simulink model "CM020A_Bmw5441McuCfg"  (R2013b)
settings: Solver=FixedStepDiscrete  SolverMode=SingleTasking  StartTime=0.0  StopTime=1  FixedStep=0.0005  RelTol=1e-3
PreLoadFcn:
  | CM020A_Bmw5441McuCfg_DataDict
values from neighbouring files (symbols this model uses):
  ADC0CFGANDUSE_ADCD0SGVCEP2_CNT_U08 = DataDict.Constant    [CM020A_Bmw5441McuCfg_DataDict.m]
  ADC0CFGANDUSE_ADCD0SGVCEP3_CNT_U08 = DataDict.Constant    [CM020A_Bmw5441McuCfg_DataDict.m]
  ADC0CFGANDUSE_ADCD0SGVCSP2_CNT_U08 = DataDict.Constant    [CM020A_Bmw5441McuCfg_DataDict.m]
  ADC0CFGANDUSE_ADCD0SGVCSP3_CNT_U08 = DataDict.Constant    [CM020A_Bmw5441McuCfg_DataDict.m]
  ADC0CFGANDUSE_ADCD0VCR00_CNT_U32 = DataDict.Constant    [CM020A_Bmw5441McuCfg_DataDict.m]
  ADC0CFGANDUSE_ADCD0VCR01_CNT_U32 = DataDict.Constant    [CM020A_Bmw5441McuCfg_DataDict.m]
  ADC0CFGANDUSE_ADCD0VCR02_CNT_U32 = DataDict.Constant    [CM020A_Bmw5441McuCfg_DataDict.m]
  ADC0CFGANDUSE_ADCD0VCR03_CNT_U32 = DataDict.Constant    [CM020A_Bmw5441McuCfg_DataDict.m]
  ADC0CFGANDUSE_ADCD0VCR04_CNT_U32 = DataDict.Constant    [CM020A_Bmw5441McuCfg_DataDict.m]
  ADC0CFGANDUSE_ADCD0VCR05_CNT_U32 = DataDict.Constant    [CM020A_Bmw5441McuCfg_DataDict.m]
  ADC0CFGANDUSE_ADCD0VCR06_CNT_U32 = DataDict.Constant    [CM020A_Bmw5441McuCfg_DataDict.m]
  ADC0CFGANDUSE_ADCD0VCR07_CNT_U32 = DataDict.Constant    [CM020A_Bmw5441McuCfg_DataDict.m]
  ADC0CFGANDUSE_ADCD0VCR08_CNT_U32 = DataDict.Constant    [CM020A_Bmw5441McuCfg_DataDict.m]
  ADC0CFGANDUSE_ADCD0VCR09_CNT_U32 = DataDict.Constant    [CM020A_Bmw5441McuCfg_DataDict.m]
  ADC0CFGANDUSE_ADCD0VCR10_CNT_U32 = DataDict.Constant    [CM020A_Bmw5441McuCfg_DataDict.m]
  ADC0CFGANDUSE_ADCD0VCR11_CNT_U32 = DataDict.Constant    [CM020A_Bmw5441McuCfg_DataDict.m]
  ADC0CFGANDUSE_ADCD0VCR12_CNT_U32 = DataDict.Constant    [CM020A_Bmw5441McuCfg_DataDict.m]
  ADC0CFGANDUSE_ADCD0VCR13_CNT_U32 = DataDict.Constant    [CM020A_Bmw5441McuCfg_DataDict.m]
  ADC0CFGANDUSE_ADCD0VCR14_CNT_U32 = DataDict.Constant    [CM020A_Bmw5441McuCfg_DataDict.m]
  ADC0CFGANDUSE_ADCD0VCR15_CNT_U32 = DataDict.Constant    [CM020A_Bmw5441McuCfg_DataDict.m]
  ADC0CFGANDUSE_ADCD0VCR16_CNT_U32 = DataDict.Constant    [CM020A_Bmw5441McuCfg_DataDict.m]
  ADC0CFGANDUSE_ADCD0VCR17_CNT_U32 = DataDict.Constant    [CM020A_Bmw5441McuCfg_DataDict.m]
  ADC0CFGANDUSE_ADCD0VCR18_CNT_U32 = DataDict.Constant    [CM020A_Bmw5441McuCfg_DataDict.m]
  ADC0CFGANDUSE_ADCD0VCR19_CNT_U32 = DataDict.Constant    [CM020A_Bmw5441McuCfg_DataDict.m]
  ADC0CFGANDUSE_ADCD0VCR20_CNT_U32 = DataDict.Constant    [CM020A_Bmw5441McuCfg_DataDict.m]
  ADC0CFGANDUSE_ADCSCAGFAC_VOLTPERCNT_F32 = DataDict.Constant    [CM020A_Bmw5441McuCfg_DataDict.m]
  ADC1CFGANDUSE_ADCD1SGVCEP2_CNT_U08 = DataDict.Constant    [CM020A_Bmw5441McuCfg_DataDict.m]
  ADC1CFGANDUSE_ADCD1SGVCEP3_CNT_U08 = DataDict.Constant    [CM020A_Bmw5441McuCfg_DataDict.m]
  ADC1CFGANDUSE_ADCD1SGVCSP2_CNT_U08 = DataDict.Constant    [CM020A_Bmw5441McuCfg_DataDict.m]
  ADC1CFGANDUSE_ADCD1SGVCSP3_CNT_U08 = DataDict.Constant    [CM020A_Bmw5441McuCfg_DataDict.m]
  ADC1CFGANDUSE_ADCD1VCR00_CNT_U32 = DataDict.Constant    [CM020A_Bmw5441McuCfg_DataDict.m]
  ADC1CFGANDUSE_ADCD1VCR01_CNT_U32 = DataDict.Constant    [CM020A_Bmw5441McuCfg_DataDict.m]
  ADC1CFGANDUSE_ADCD1VCR02_CNT_U32 = DataDict.Constant    [CM020A_Bmw5441McuCfg_DataDict.m]
  ADC1CFGANDUSE_ADCD1VCR03_CNT_U32 = DataDict.Constant    [CM020A_Bmw5441McuCfg_DataDict.m]
  ADC1CFGANDUSE_ADCD1VCR04_CNT_U32 = DataDict.Constant    [CM020A_Bmw5441McuCfg_DataDict.m]
  ADC1CFGANDUSE_ADCD1VCR05_CNT_U32 = DataDict.Constant    [CM020A_Bmw5441McuCfg_DataDict.m]
  ADC1CFGANDUSE_ADCD1VCR06_CNT_U32 = DataDict.Constant    [CM020A_Bmw5441McuCfg_DataDict.m]
  ADC1CFGANDUSE_ADCD1VCR07_CNT_U32 = DataDict.Constant    [CM020A_Bmw5441McuCfg_DataDict.m]
  ADC1CFGANDUSE_ADCD1VCR08_CNT_U32 = DataDict.Constant    [CM020A_Bmw5441McuCfg_DataDict.m]
  ADC1CFGANDUSE_ADCD1VCR09_CNT_U32 = DataDict.Constant    [CM020A_Bmw5441McuCfg_DataDict.m]
  ADC1CFGANDUSE_ADCD1VCR10_CNT_U32 = DataDict.Constant    [CM020A_Bmw5441McuCfg_DataDict.m]
  ADC1CFGANDUSE_ADCD1VCR11_CNT_U32 = DataDict.Constant    [CM020A_Bmw5441McuCfg_DataDict.m]
  ADC1CFGANDUSE_ADCD1VCR12_CNT_U32 = DataDict.Constant    [CM020A_Bmw5441McuCfg_DataDict.m]
  ADC1CFGANDUSE_ADCD1VCR13_CNT_U32 = DataDict.Constant    [CM020A_Bmw5441McuCfg_DataDict.m]
  ADC1CFGANDUSE_ADCD1VCR14_CNT_U32 = DataDict.Constant    [CM020A_Bmw5441McuCfg_DataDict.m]
  ADC1CFGANDUSE_ADCD1VCR15_CNT_U32 = DataDict.Constant    [CM020A_Bmw5441McuCfg_DataDict.m]
  ADC1CFGANDUSE_ADCD1VCR16_CNT_U32 = DataDict.Constant    [CM020A_Bmw5441McuCfg_DataDict.m]
  ADC1CFGANDUSE_ADCD1VCR17_CNT_U32 = DataDict.Constant    [CM020A_Bmw5441McuCfg_DataDict.m]
  ADC1CFGANDUSE_ADCD1VCR18_CNT_U32 = DataDict.Constant    [CM020A_Bmw5441McuCfg_DataDict.m]
  ADC1CFGANDUSE_ADCD1VCR19_CNT_U32 = DataDict.Constant    [CM020A_Bmw5441McuCfg_DataDict.m]
  ADC1CFGANDUSE_ADCD1VCR20_CNT_U32 = DataDict.Constant    [CM020A_Bmw5441McuCfg_DataDict.m]
  ADCDIAGC_DYNDIAGFAILSTEP_CNT_U16 = DataDict.Constant    [CM020A_Bmw5441McuCfg_DataDict.m]
  ADCDIAGC_DYNDIAGPASSSTEP_CNT_U16 = DataDict.Constant    [CM020A_Bmw5441McuCfg_DataDict.m]
  BATTRTNCURR_CURRESTIMDIFTHD_AMPR_F32 = DataDict.Constant    [CM020A_Bmw5441McuCfg_DataDict.m]
  BATTRTNCURR_FAILSTEP_CNT_U16 = DataDict.Constant    [CM020A_Bmw5441McuCfg_DataDict.m]
  BATTRTNCURR_FASTLOOPPROC_CNT_LOGL = DataDict.Constant    [CM020A_Bmw5441McuCfg_DataDict.m]
  BATTRTNCURR_FILCUTFREQ_HZ_F32 = DataDict.Constant    [CM020A_Bmw5441McuCfg_DataDict.m]
  BATTRTNCURR_GAIN_AMPRPERVOLT_F32 = DataDict.Constant    [CM020A_Bmw5441McuCfg_DataDict.m]
  BATTRTNCURR_LOWRTHD_AMPR_F32 = DataDict.Constant    [CM020A_Bmw5441McuCfg_DataDict.m]
  BATTRTNCURR_OFFSET_VOLT_F32 = DataDict.Constant    [CM020A_Bmw5441McuCfg_DataDict.m]
  BATTRTNCURR_OUTPMAX_AMPR_F32 = DataDict.Constant    [CM020A_Bmw5441McuCfg_DataDict.m]
  BATTRTNCURR_OUTPMIN_AMPR_F32 = DataDict.Constant    [CM020A_Bmw5441McuCfg_DataDict.m]
  BATTRTNCURR_PASSSTEP_CNT_U16 = DataDict.Constant    [CM020A_Bmw5441McuCfg_DataDict.m]
  BATTRTNCURR_UPPRTHD_AMPR_F32 = DataDict.Constant    [CM020A_Bmw5441McuCfg_DataDict.m]
  BATTVLTGSCAGFAC_ULS_F32 = DataDict.Constant    [CM020A_Bmw5441McuCfg_DataDict.m]
  BATTVLTGSWD1SCAGFAC_ULS_F32 = DataDict.Constant    [CM020A_Bmw5441McuCfg_DataDict.m]
  ECUTMEAS_DFTT_DEGCGRD_F32 = DataDict.Constant    [CM020A_Bmw5441McuCfg_DataDict.m]
  ECUTMEAS_ECUTX_VOLT_U3P13 = DataDict.Constant    [CM020A_Bmw5441McuCfg_DataDict.m]
  ECUTMEAS_ECUTY_DEGCGRD_S8P7 = DataDict.Constant    [CM020A_Bmw5441McuCfg_DataDict.m]
  ECUTMEAS_FILTAU_HZ_F32 = DataDict.Constant    [CM020A_Bmw5441McuCfg_DataDict.m]
  ECUTMEAS_NTC0X045FAILSTEP_CNT_U16 = DataDict.Constant    [CM020A_Bmw5441McuCfg_DataDict.m]
  ECUTMEAS_NTC0X045PASSSTEP_CNT_U16 = DataDict.Constant    [CM020A_Bmw5441McuCfg_DataDict.m]
  ECUTMEAS_RNGDIAGCMAX_DEGCGRD_F32 = DataDict.Constant    [CM020A_Bmw5441McuCfg_DataDict.m]
  ECUTMEAS_RNGDIAGCMIN_DEGCGRD_F32 = DataDict.Constant    [CM020A_Bmw5441McuCfg_DataDict.m]
  ELECGLBPRM_IVTRCNT_CNT_U08 = DataDict.Constant    [CM020A_Bmw5441McuCfg_DataDict.m]
  ELECGLBPRM_PWMFRQMAX_HZ_U32 = DataDict.Constant    [CM020A_Bmw5441McuCfg_DataDict.m]
  ELECGLBPRM_PWMFRQMIN_HZ_U32 = DataDict.Constant    [CM020A_Bmw5441McuCfg_DataDict.m]
  ELECGLBPRM_PWMPERDMAX_NANOSEC_U32 = DataDict.Constant    [CM020A_Bmw5441McuCfg_DataDict.m]
  ELECGLBPRM_PWMPERDMIN_NANOSEC_U32 = DataDict.Constant    [CM020A_Bmw5441McuCfg_DataDict.m]
  ELECGLBPRM_PWMPERDNOM_MICROSEC_U7P9 = DataDict.Constant    [CM020A_Bmw5441McuCfg_DataDict.m]
  ELECGLBPRM_PWMPERDNOMX2_SEC_F32 = DataDict.Constant    [CM020A_Bmw5441McuCfg_DataDict.m]
  FLTINJENA = DataDict.Constant    [CM020A_Bmw5441McuCfg_DataDict.m]
  HWTQ4MEAS_HWTQ4RNGCHKPRTCLNTCNR_CNT_ENUM = DataDict.Constant    [CM020A_Bmw5441McuCfg_DataDict.m]
  HWTQ4MEAS_HWTQ4SCANOTPRFMMFGNTCNR_CNT_ENUM = DataDict.Constant    [CM020A_Bmw5441McuCfg_DataDict.m]
  HWTQ4MEAS_HWTQ4TRIMNOTPRFMMFGNTCNR_CNT_ENUM = DataDict.Constant    [CM020A_Bmw5441McuCfg_DataDict.m]
  HWTQ4MEAS_HWTQBARSTFN_NMPDEG_F32 = DataDict.Constant    [CM020A_Bmw5441McuCfg_DataDict.m]
  HWTQ4MEAS_HWTQOFFS_VOLT_F32 = DataDict.Constant    [CM020A_Bmw5441McuCfg_DataDict.m]
  HWTQ4MEAS_HWTQSNSRSCANOMVAL_VOLTPDEG_F32 = DataDict.Constant    [CM020A_Bmw5441McuCfg_DataDict.m]
  HWTQ5MEAS_HWTQ5RNGCHKPRTCLNTCNR_CNT_ENUM = DataDict.Constant    [CM020A_Bmw5441McuCfg_DataDict.m]
  HWTQ5MEAS_HWTQ5SCANOTPRFMMFGNTCNR_CNT_ENUM = DataDict.Constant    [CM020A_Bmw5441McuCfg_DataDict.m]
  HWTQ5MEAS_HWTQ5TRIMNOTPRFMMFGNTCNR_CNT_ENUM = DataDict.Constant    [CM020A_Bmw5441McuCfg_DataDict.m]
  HWTQ5MEAS_HWTQBARSTFN_NMPDEG_F32 = DataDict.Constant    [CM020A_Bmw5441McuCfg_DataDict.m]
  HWTQ5MEAS_HWTQOFFS_VOLT_F32 = DataDict.Constant    [CM020A_Bmw5441McuCfg_DataDict.m]
  HWTQ5MEAS_HWTQSNSRSCANOMVAL_VOLTPDEG_F32 = DataDict.Constant    [CM020A_Bmw5441McuCfg_DataDict.m]
  MOTAG0MEAS_MOTAG0PRTCLFLTNTCNR_CNT_ENUM = DataDict.Constant    [CM020A_Bmw5441McuCfg_DataDict.m]
  MOTAG1MEAS_MOTAG1PRTCLFLTNTCNR_CNT_ENUM = DataDict.Constant    [CM020A_Bmw5441McuCfg_DataDict.m]
  MOTAG3MEAS_SNSRRLVBITWIDTHEXP_CNT_U08 = DataDict.Constant    [CM020A_Bmw5441McuCfg_DataDict.m]
  MOTAG4MEAS_SNSRRLVBITWIDTHEXP_CNT_U08 = DataDict.Constant    [CM020A_Bmw5441McuCfg_DataDict.m]
  RVSBATTPROTN_FAILSTEP_CNT_U16 = DataDict.Constant    [CM020A_Bmw5441McuCfg_DataDict.m]
  RVSBATTPROTN_GNDMEASDVLTGHILIMN_VOLT_F32 = DataDict.Constant    [CM020A_Bmw5441McuCfg_DataDict.m]
  RVSBATTPROTN_GNDMEASDVLTGLOLIMN_VOLT_F32 = DataDict.Constant    [CM020A_Bmw5441McuCfg_DataDict.m]
  RVSBATTPROTN_PASSSTEP_CNT_U16 = DataDict.Constant    [CM020A_Bmw5441McuCfg_DataDict.m]
  RVSBATTPROTN_RTNMEASDVLTGHILIMN_VOLT_F32 = DataDict.Constant    [CM020A_Bmw5441McuCfg_DataDict.m]
  RVSBATTPROTN_RTNMEASDVLTGLOLIMN_VOLT_F32 = DataDict.Constant    [CM020A_Bmw5441McuCfg_DataDict.m]
  RVSBATTPROTN_RVSFLTTHD_VOLT_F32 = DataDict.Constant    [CM020A_Bmw5441McuCfg_DataDict.m]
  SWPENA = DataDict.Constant    [CM020A_Bmw5441McuCfg_DataDict.m]
  TUNSELNAUTHY_XCPVEHSPDTHD_KPH_F32 = DataDict.Constant    [CM020A_Bmw5441McuCfg_DataDict.m]
libraries: CM020A_Bmw5441McuCfg_ModelLibrary x82, simulink x24
(part 1 of 3)
settings Model: Creator=nz3zln  LastModifiedBy=TZBSJD
settings SolverCC: AutoInsertRateTranBlk=on  InsertRTBMode=Always
settings DataIOCC: LimitDataPoints=off  SaveFormat=Structure  ReturnWorkspaceOutputs=on
settings OptimizationCC: BlockReduction=off  InlineParams=on  ZeroExternalMemoryAtStartup=off  ZeroInternalMemoryAtStartup=off  OptimizeModelRefInitCode=on  LifeSpan=1
settings DebuggingCC: SignalInfNanChecking=error  SignalRangeChecking=warning  UnderspecifiedInitializationDetection=Simplified  SolverPrmCheckMsg=error  InheritedTsInSrcMsg=error  DiscreteInheritContinuousMsg=error  SingleTaskRateTransMsg=error  TasksWithSamePriorityMsg=error  SigSpecEnsureSampleTimeMsg=error  CheckMatrixSingularityMsg=error  ParameterUnderflowMsg=error  ParameterPrecisionLossMsg=error  ParameterTunabilityLossMsg=error  FixptConstUnderflowMsg=warning  FixptConstOverflowMsg=warning  VectorMatrixConversionMsg=error  SignalLabelMismatchMsg=error  UnconnectedInputMsg=error  UnconnectedOutputMsg=error  UnconnectedLineMsg=error  SFcnCompatibilityMsg=error  UniqueDataStoreMsg=warning  BusObjectLabelMismatch=error  RootOutportRequireBusObject=error  AssertControl=DisableAll  ModelReferenceIOMsg=error  ModelReferenceVersionMismatchMessage=warning  ModelReferenceIOMismatchMessage=error  ModelReferenceCSMismatchMessage=warning  ModelReferenceDataLoggingMessage=error  StateNameClashWarn=warning  StrictBusMsg=ErrorOnBusTreatedAsVector  NonBusSignalsTreatedAsBus=error  SFUnexpectedBacktrackingDiag=error  SFInvalidInputDataAccessInChartInitDiag=error  SFNoUnconditionalDefaultTransitionDiag=error  SFTransitionOutsideNaturalParentDiag=error  SFUnconditionalTransitionShadowingDiag=error  SFUndirectedBroadcastEventsDiag=error
settings ModelReferenceCC: ModelReferenceNumInstancesAllowed=Single
settings RTWCC: SystemTargetFile=autosar.tlc  GenCodeOnly=on  TemplateMakefile=ert_default_tmf  Description=AUTOSAR  GenerateReport=on  ProcessScript=autosar_make_rtw_hook  LaunchReport=on
settings CodeAppCC: GenerateComments=off  IgnoreCustomStorageClasses=off  CustomSymbolStrType=$N$R$M  CustomSymbolStrBlkIO=$N$M  SimulinkBlockComments=off
settings STFCustomTargetCC: ParMdlRefBuildCompliant=on  CompOptLevelCompliant=on  IncludeMdlTerminateFcn=off  CombineOutputUpdateFcns=on  SuppressErrorStatus=on  ERTFirstTimeCompliant=on  ERTCustomFileBanners=on  SupportNonFinite=off  SupportComplex=off  SupportContinuousTime=off  SupportNonInlinedSFcns=off  MATLABClassNameForMDSCustomization=Simulink.SoftwareTarget.ERTCustomization  AutosarCompliant=on  GRTInterface=off  SystemTargetFile=autosar.tlc
settings ERTTargetCC: CodeReplacementLibrary=ANSI_C  ConcurrentExecutionCompliant=off  IncludeMdlTerminateFcn=off  SuppressErrorStatus=on  SupportNonFinite=off  SupportComplex=off  ModelStepFunctionPrototypeControlCompliant=off  CPPClassGenCompliant=off  AutosarCompliant=on  InlinedParameterPlacement=NonHierarchical  ERTCustomFileTemplate=example_file_process.tlc  EnableUserReplacementTypes=on

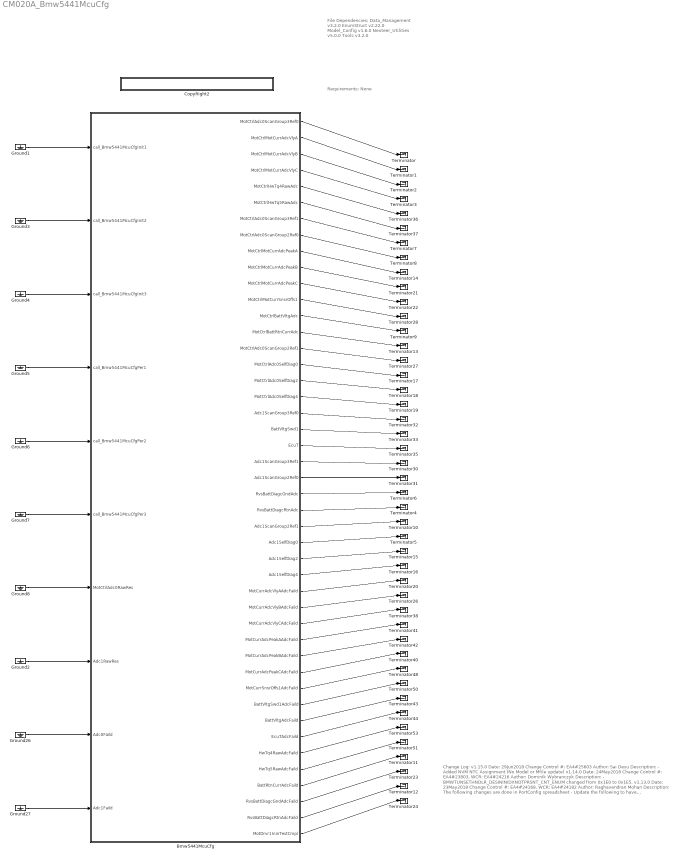
== system CM020A_Bmw5441McuCfg ==
  note: File Dependencies:
      |
      | Data_Management v3.2.0
      | EnumStruct v2.22.0
      | Model_Config v1.6.0
      | Nexteer_Utilities v5.0.0
      | Tools v3.2.0
  note: Change Log:
      |
      | v1.15.0
      | Date: 29Jun2018
      | Change Control #: EA4#25603
      | Author: Sai Desu
      | Description:
      | - Added NVM NTC Assignment (No Model or Mfile update)
      |
      |
      | v1.14.0
      | Date: 24May2018
      | Change Control #: EA4#23803, WCR: EA4#24216
      | Author: Dominik Wybranczyk
      | Description:
      | - BMWTUNSETHNDLR_DESININIDXNOTPRSNT_CNT_ENUM changed from 0x1E0 to 0x1E5.
      |
      |
      | v1.13.0
      | Date: 23May2018
      | Change Control #: EA4#24168, WCR: EA4#24182
      | Author: Raghavendran Mohan
      | Description:
      | The following changes are done in PortConfig spreadsheet
      | - Update the following to have PortPinDioAltModeChangeable = TRUE
      | 	Port_PortGroup2_PortPin8_MotAg0Mosi
      | 	Port_PortGroup2_PortPin9_MotAg0Clk
      | 	Port_PortGroup4_PortPin3_MotAg0Cs
      | 	Port_PortGroup2_PortPin5_MotAg2Mosi
      | 	Port_PortGroup2_PortPin7_MotAg2Clk
      | 	Port_PortGroup3_PortPin3_MotAg2Cs
      | - Update MotAg2 Hardware identifier to MotAg1
      | The following changes are done in DataDict File
      | - Update EcuT X and Y table to account for NTC thresholds
      |   ECUTMEAS_ECUTY_DEGCGRD_S8P7 and
      | 	ECUTMEAS_ECUTX_VOLT_U3P13
      |
      |
      | v1.12.0
      | Date: 22May2018
      | Change Control #: EA4#24074, WCR: EA4#24076
      | Author: D.Wybranczyk
      | Description:
      | - Updating interpolation table for ECUTMEAS to match sensor characteristics (LM60)
      | 	ECUTMEAS_ECUTY_DEGCGRD_S8P7 and
      | 	ECUTMEAS_ECUTX_VOLT_U3P13
      | - Adding constants for:
      | 	BMWTUNSETHNDLR_DESININIDXNOTPRSNT_CNT_ENUM as NTCNR_0X1E0
      | 	BMWTUNSETHNDLR_DESININOPTSETAISXNOTPRSNT_CNT_ENUM as NTCNR_0X1E06
      |
      |
      | v1.11.0
      | Date: 06Mar2018
      | Change Control #: EA4#20822, EA4#21100
      | Author: Dominik Wybranczyk
      | Description:
      | - Restored ELECGLBPRM_MOTCTRLINTRPTTRIGSRC_CNT_U08 with value 0 as CM475 owner request (disable peak interrupt generation)
      | - Enabled Inverter Fet Fault Mitigation reporting with GATEDRV0FETFLTMTGTNENA_ULS_LOGL = 1
      | - Changed Reverse Battery Protection - Reverse Threshold value RVSBATTPROTN_RVSFLTTHD_VOLT_F32 from 0.4 to 0.6
      |
      |
      | v1.10.0
      | Date: 04Jan2018
      | Change Control #: EA4#9561, 	EA4#17983.
      | Author: Dominik Wybranczyk
      | Description:
      | - Deleted Motor Control Interrupt Trigger Source constant ELECGLBPRM_MOTCTRLINTRPTTRIGSRC_CNT_U08 (not needed)
      | - Updated HwTq naming convention in PortConfig and in the model.
      | - Enabled TAUJ Filter for pins 20,21,23 in new file DigitalNoiseFilterConfig.xlsx
      | - Unification of Constant definitions (changed to 'Local').
      | - Introduced configuration tables (Constants) for Diagnostic Manager
      | 	DIAGCMGRLISTOFLTCHGNTC_CNT_ENUM and DIAGCMGRNTCLTCHCNTRTHD_CNT_U08.
      | - Introduced constants GATEDRV0FETFLTMTGTNENA_ULS_LOGL, MCUDIAGCERRINJ.
      | - Updated TUNSELNAUTHY_XCPVEHSPDTHD_KPH_F32 dataType.
      |
      | v1.9.0
      | Date: 22Nov2017
      | Change Control #: EA4#17722
      | Author: Dominik Wybranczyk
      | Description:
      | - PortConfig Update for MISO and CLK pins for CSIH1, CSIH2 and CSIH3.
      | - Introduced new constants APPLCRCREGNNR_CNT_U08
      | 	and ELECGLBPRM_MOTCTRLINTRPTTRIGSRC_CNT_U08.
      |
      | v1.8.0
      | Date: 10Nov2017
      | Change Control #: EA4#14956, WCR: EA4#17309
      | Author: Dominik Wybranczyk
      | Description:
      | - QEP Interface PortConfig modification (for index pin).
      | - New constants for  CM510A and CM515A.
      | - Update to RegisterConfiguration for ENCA.
      | - No functional change in the model
      |
      | v1.7.0
      | Date: 25Oct2017
      | Change Control #: EA4#14956, WCR: EA4#16383
      | Author: Dominik Wybranczyk
      | Description:
      | - New configuration for QEP interface (ABI) in PortConfig
      | - New output in Per3: MotDrvr1IninTestCmpl
      |
      | v1.6.0
      | Date: 12Oct2017
      | Change Control #: EA4#16147 & EA4#14904
      | Author: Dominik Wybranczyk
      | Description:
      | - Added and updated constants for ES251A in DataDict.
      | - Added constants for ES252 in DataDict.
      | - No functional changes in the model.
      | - Update to PortConfig for pins P2_3, P2_15, P3_4, P4_11, P5_3.
      |
      | v1.5.0
      | Date: 11Oct2017
      | Change Control #: EA4#16075
      | Author: Dominik Wybranczyk
      | - Change to constants values for ES210A in DataDict.
      | - No functional change in the model.
      |
      | v1.4.0
      | Date: 02Oct2017
      | Change Control #: WCR: EA4#15646; PCR: EA4#15645
      | Author: Dominik Wybranczyk
      | Description:
      | - Added ES210A ConfigParams as Constants.
      | - Change Log clarification update.
      |
      |
      | Version		1.3.0
      | Date		26Jul2017
      | Change Control#: EA4#14071
      | Modified By:	Dominik Wybranczyk
      | Changes:
      | - Add ConfigParam from ES251A. Signal name fix.
      |
      |
      | Version		1.2.0
      | Date		27Jun2017
      | Change Control#: EA4#13327
      | Modified By:	Dominik Wybranczyk
      | Changes:
      | - Modified design for new board release and I185.
      | - Changed configuration for single inverter.
      | - Deleted signals connected with phase D, E and F.
      | - Changed PortConfiguration.
      | - Changed AdcConfiguration.
      | - Clarification improvements.
      |
      |
      | Version		1.1.0
      | Date 		22DEC2016
      | Modified By: 	J. Erlenbeck
      | Changes		Moved to dual inverter, substantial ADC configuration changes
      |
      |
      | Version		1.0.0
      | Date
      | Modified By: 	J. Erlenbeck
      | Changes		Initial Release
  note: Requirements:
      |
      | None
  Bmw5441McuCfg : Subsystem
  CopyRight2 : Subsystem  Description=|  mask(Copyright Information){none=on}
      | Copyright info block.                                               
      |                                                                     
      | Place copyright information at the top of every subsystem in design.
      mask prompts: none "No parameters"
      mask help: Place copyright information at the top of every subsystem in design.
      mask Display:
      | NxtrConf = 'Nexteer Confidential';
      | 
      | sys = bdroot; %handle for the current model ("system")
      | first = get_param(sys,'Created');
      | first = first(end-3:end);  %year is last four digits
      | 
      | last = get_param(sys,'LastModifiedDate');
      | if isempty(last)
      |     last = datestr(now,'yyyy');
      | else
      |     last = last(end-3:end);
      | end
      | 
      | if strcmp(first,last)
      |     fprintf('%s -- Copyright %s Nexteer',NxtrConf,first)
      | else
      |     fprintf('%s -- %s%s- %s Nexteer',NxtrConf,char(169),first,last)
      | end
  Ground{1..8,26..27} (10 alike) : Ground
  Terminator{,1..24,26..28,30..33,35..38,40..44,48,50..51,53} (45 alike) : Terminator
  wires:
  Ground26/1 -> Bmw5441McuCfg/9(Adc0Faild)
  Ground27/1 -> Bmw5441McuCfg/10(Adc1Faild)
  Bmw5441McuCfg/1(MotCtrlAdc0ScanGroup3Ref0) -> Terminator/1
  Bmw5441McuCfg/2(MotCtrlMotCurrAdcVlyA) -> Terminator1/1
  Bmw5441McuCfg/3(MotCtrlMotCurrAdcVlyB) -> Terminator2/1
  Bmw5441McuCfg/4(MotCtrlMotCurrAdcVlyC) -> Terminator3/1
  Bmw5441McuCfg/7(MotCtrlAdc0ScanGroup3Ref1) -> Terminator7/1
  Bmw5441McuCfg/8(MotCtrlAdc0ScanGroup2Ref0) -> Terminator8/1
  Bmw5441McuCfg/16(MotCtrlAdc0SelfDiag0) -> Terminator17/1
  Bmw5441McuCfg/17(MotCtrlAdc0SelfDiag2) -> Terminator18/1
  Bmw5441McuCfg/18(MotCtrlAdc0SelfDiag4) -> Terminator19/1
  Bmw5441McuCfg/9(MotCtrlMotCurrAdcPeakA) -> Terminator14/1
  Bmw5441McuCfg/10(MotCtrlMotCurrAdcPeakB) -> Terminator21/1
  Bmw5441McuCfg/11(MotCtrlMotCurrAdcPeakC) -> Terminator22/1
  Bmw5441McuCfg/12(MotCtrlMotCurrSnsrOffs1) -> Terminator28/1
  Bmw5441McuCfg/15(MotCtrlAdc0ScanGroup2Ref1) -> Terminator27/1
  Bmw5441McuCfg/19(Adc1ScanGroup3Ref0) -> Terminator32/1
  Bmw5441McuCfg/20(BattVltgSwd1) -> Terminator33/1
  Bmw5441McuCfg/21(EcuT) -> Terminator35/1
  Bmw5441McuCfg/5(MotCtrlHwTq4RawAdc) -> Terminator36/1
  Bmw5441McuCfg/6(MotCtrlHwTq5RawAdc) -> Terminator37/1
  Bmw5441McuCfg/22(Adc1ScanGroup3Ref1) -> Terminator30/1
  Bmw5441McuCfg/23(Adc1ScanGroup2Ref0) -> Terminator31/1
  Bmw5441McuCfg/13(MotCtrlBattVltgAdc) -> Terminator9/1
  Bmw5441McuCfg/26(Adc1ScanGroup2Ref1) -> Terminator10/1
  Bmw5441McuCfg/27(Adc1SelfDiag0) -> Terminator5/1
  Bmw5441McuCfg/28(Adc1SelfDiag2) -> Terminator15/1
  Bmw5441McuCfg/29(Adc1SelfDiag4) -> Terminator16/1
  Bmw5441McuCfg/30(MotCurrAdcVlyAAdcFaild) -> Terminator20/1
  Bmw5441McuCfg/31(MotCurrAdcVlyBAdcFaild) -> Terminator26/1
  Bmw5441McuCfg/32(MotCurrAdcVlyCAdcFaild) -> Terminator38/1
  Bmw5441McuCfg/33(MotCurrAdcPeakAAdcFaild) -> Terminator41/1
  Bmw5441McuCfg/34(MotCurrAdcPeakBAdcFaild) -> Terminator42/1
  Bmw5441McuCfg/35(MotCurrAdcPeakCAdcFaild) -> Terminator40/1
  Bmw5441McuCfg/36(MotCurrSnsrOffs1AdcFaild) -> Terminator48/1
  Bmw5441McuCfg/37(BattVltgSwd1AdcFaild) -> Terminator50/1
  Bmw5441McuCfg/38(BattVltgAdcFaild) -> Terminator43/1
  Bmw5441McuCfg/39(EcuTAdcFaild) -> Terminator44/1
  Bmw5441McuCfg/40(HwTq4RawAdcFaild) -> Terminator53/1
  Bmw5441McuCfg/41(HwTq5RawAdcFaild) -> Terminator51/1
  Bmw5441McuCfg/24(RvsBattDiagcGndAdc) -> Terminator6/1
  Bmw5441McuCfg/25(RvsBattDiagcRtnAdc) -> Terminator4/1
  Bmw5441McuCfg/14(MotCtrlBattRtnCurrAdc) -> Terminator13/1
  Bmw5441McuCfg/42(BattRtnCurrAdcFaild) -> Terminator11/1
  Bmw5441McuCfg/43(RvsBattDiagcGndAdcFaild) -> Terminator23/1
  Bmw5441McuCfg/44(RvsBattDiagcRtnAdcFaild) -> Terminator12/1
  Ground2/1 -> Bmw5441McuCfg/8(Adc1RawRes)
  Ground1/1 -> Bmw5441McuCfg/1(call_Bmw5441McuCfgInit1)
  Ground3/1 -> Bmw5441McuCfg/2(call_Bmw5441McuCfgInit2)
  Ground4/1 -> Bmw5441McuCfg/3(call_Bmw5441McuCfgInit3)
  Ground5/1 -> Bmw5441McuCfg/4(call_Bmw5441McuCfgPer1)
  Ground6/1 -> Bmw5441McuCfg/5(call_Bmw5441McuCfgPer2)
  Ground7/1 -> Bmw5441McuCfg/6(call_Bmw5441McuCfgPer3)
  Ground8/1 -> Bmw5441McuCfg/7(MotCtrlAdc0RawRes)
  Bmw5441McuCfg/45(MotDrvr1IninTestCmpl) -> Terminator24/1

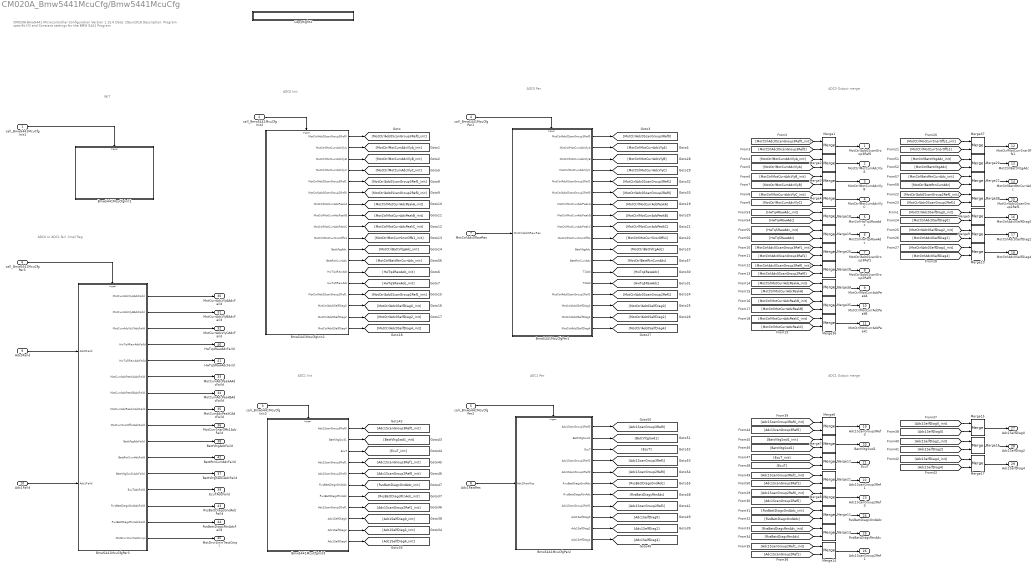
== system CM020A_Bmw5441McuCfg/Bmw5441McuCfg ==
  note: ADC1 Init
  note: CM020A Bmw5441 Microcontroller Configuration
      |
      | Version 1.15.0
      | Date: 29Jun2018
      |
      | Description:
      | Program specific I/O and Constant settings for the BMW 5441 Program
  note: ADC0 Init
  note: ADC0 or ADC1 fail, Cmpl flag
  note: INIT
  note: ADC0 Per
  note: ADC0 Output merge
  note: ADC1 Per
  note: ADC1 Output merge
  call_Bmw5441McuCfgInit1 : Inport
  call_Bmw5441McuCfgInit2 : Inport  Port=2
  call_Bmw5441McuCfgInit3 : Inport  Port=3
  call_Bmw5441McuCfgPer1 : Inport  Port=4
  call_Bmw5441McuCfgPer2 : Inport  Port=5
  call_Bmw5441McuCfgPer3 : Inport  Port=6
  MotCtrlAdc0RawRes : Inport  Port=7
  Adc1RawRes : Inport  Port=8
  Adc0Faild : Inport  Port=9
  Adc1Faild : Inport  Port=10
  Bmw5441McuCfgInit1 : Subsystem  RequirementInfo="{'linktype_rmi_doors' '0000c472 (/ESG Group/FDD Module Requirements/EA4 Specific/CM300A_Adc0CfgAndUse)' '#CM300A_95' 'true' 'REQ:  CM300A_95' '' ; 'linktype_rmi_doors' '0000c475 (/ESG Group/FDD Module Requirements/EA4 Specific/CM320A_Adc1CfgAndUse)' '#CM320A_92' 'true' 'REQ:  CM320A_92' '' } %GIDa_37aeff40_c03b_483a_98dc_cda618c9a3ba"
  Bmw5441McuCfgInit2 : Subsystem  RequirementInfo="{}  %GIDa_e4555fdb_3a20_41e8_bf37_7a040ba879e8"
  Bmw5441McuCfgInit3 : Subsystem
  Bmw5441McuCfgPer1 : Subsystem  RequirementInfo={'linktype_rmi_doors' '0000c472 (/ESG Group/FDD Module Requirements/EA4 Specific/CM300A_Adc0CfgAndUse)' '#CM300A_76' 'true' 'REQ: CM300A_76' '' } %GIDa_873a1ca9_93ed_4591_b882_6d7fd3820ab2
      settings: AttributesFormatString=Priority: %<Priority>
  Bmw5441McuCfgPer2 : Subsystem  RequirementInfo="{'linktype_rmi_doors' '0000c475 (/ESG Group/FDD Module Requirements/EA4 Specific/CM320A_Adc1CfgAndUse)' '#CM320A_76' 'true' 'REQ:  CM320A_76' '' } %GIDa_f8eec309_27b4_4df0_b18c_c2951f94362c"
      settings: AttributesFormatString=Priority: %<Priority>
  Bmw5441McuCfgPer3 : Subsystem  RequirementInfo={} %GIDa_f61b09d0_e9f4_4379_bee3_c878705b543d
      settings: AttributesFormatString=Priority: %<Priority>
  CopyRight2 : Subsystem  Description=|  mask(Copyright Information){none=on}
      | Copyright info block.                                               
      |                                                                     
      | Place copyright information at the top of every subsystem in design.
      mask prompts: none "No parameters"
      mask help: Place copyright information at the top of every subsystem in design.
      mask Display:
      | NxtrConf = 'Nexteer Confidential';
      | 
      | sys = bdroot; %handle for the current model ("system")
      | first = get_param(sys,'Created');
      | first = first(end-3:end);  %year is last four digits
      | 
      | last = get_param(sys,'LastModifiedDate');
      | if isempty(last)
      |     last = datestr(now,'yyyy');
      | else
      |     last = last(end-3:end);
      | end
      | 
      | if strcmp(first,last)
      |     fprintf('%s -- Copyright %s Nexteer',NxtrConf,first)
      | else
      |     fprintf('%s -- %s%s- %s Nexteer',NxtrConf,char(169),first,last)
      | end
  Merge{1..22,26,28,34..38} (29 alike) : Merge
  MotCtrlAdc0ScanGroup3Ref0 : Outport
  MotCtrlMotCurrAdcVlyA : Outport  Port=2
  MotCtrlMotCurrAdcVlyB : Outport  Port=3
  MotCtrlMotCurrAdcVlyC : Outport  Port=4
  MotCtrlHwTq4RawAdc : Outport  Port=5
  MotCtrlHwTq5RawAdc : Outport  Port=6
  MotCtrlAdc0ScanGroup3Ref1 : Outport  Port=7
  MotCtrlAdc0ScanGroup2Ref0 : Outport  Port=8
  MotCtrlMotCurrAdcPeakA : Outport  Port=9
  MotCtrlMotCurrAdcPeakB : Outport  Port=10
  MotCtrlMotCurrAdcPeakC : Outport  Port=11
  MotCtrlMotCurrSnsrOffs1 : Outport  Port=12
  MotCtrlBattVltgAdc : Outport  Port=13
  MotCtrlBattRtnCurrAdc : Outport  Port=14
  MotCtrlAdc0ScanGroup2Ref1 : Outport  Port=15
  MotCtrlAdc0SelfDiag0 : Outport  Port=16
  MotCtrlAdc0SelfDiag2 : Outport  Port=17
  MotCtrlAdc0SelfDiag4 : Outport  Port=18
  Adc1ScanGroup3Ref0 : Outport  Port=19
  BattVltgSwd1 : Outport  Port=20
  EcuT : Outport  Port=21
  Adc1ScanGroup3Ref1 : Outport  Port=22
  Adc1ScanGroup2Ref0 : Outport  Port=23
  RvsBattDiagcGndAdc : Outport  Port=24
  RvsBattDiagcRtnAdc : Outport  Port=25
  Adc1ScanGroup2Ref1 : Outport  Port=26
  Adc1SelfDiag0 : Outport  Port=27
  Adc1SelfDiag2 : Outport  Port=28
  Adc1SelfDiag4 : Outport  Port=29
  MotCurrAdcVlyAAdcFaild : Outport  Port=30
  MotCurrAdcVlyBAdcFaild : Outport  Port=31
  MotCurrAdcVlyCAdcFaild : Outport  Port=32
  MotCurrAdcPeakAAdcFaild : Outport  Port=33
  MotCurrAdcPeakBAdcFaild : Outport  Port=34
  MotCurrAdcPeakCAdcFaild : Outport  Port=35
  MotCurrSnsrOffs1AdcFaild : Outport  Port=36
  BattVltgSwd1AdcFaild : Outport  Port=37
  BattVltgAdcFaild : Outport  Port=38
  EcuTAdcFaild : Outport  Port=39
  HwTq4RawAdcFaild : Outport  Port=40
  HwTq5RawAdcFaild : Outport  Port=41
  BattRtnCurrAdcFaild : Outport  Port=42
  RvsBattDiagcGndAdcFaild : Outport  Port=43
  RvsBattDiagcRtnAdcFaild : Outport  Port=44
  MotDrvr1IninTestCmpl : Outport  Port=45
  wires:
  call_Bmw5441McuCfgPer1/1 -> Bmw5441McuCfgPer1/Trigger
  call_Bmw5441McuCfgPer2/1 -> Bmw5441McuCfgPer2/Trigger
  call_Bmw5441McuCfgInit1/1 -> Bmw5441McuCfgInit1/Trigger
  MotCtrlAdc0RawRes/1 -> Bmw5441McuCfgPer1/1(MotCtrlAdc0RawRes)
  Adc1RawRes/1 -> Bmw5441McuCfgPer2/1(Adc1RawRes)
  call_Bmw5441McuCfgPer3/1 -> Bmw5441McuCfgPer3/Trigger
  Adc0Faild/1 -> Bmw5441McuCfgPer3/1(Adc0Faild)
  Adc1Faild/1 -> Bmw5441McuCfgPer3/2(Adc1Faild)
  call_Bmw5441McuCfgInit2/1 -> Bmw5441McuCfgInit2/Trigger
  call_Bmw5441McuCfgInit3/1 -> Bmw5441McuCfgInit3/Trigger
  Merge1/1 -> MotCtrlAdc0ScanGroup3Ref0/1
  Merge2/1 -> MotCtrlMotCurrAdcVlyA/1
  Merge3/1 -> MotCtrlMotCurrAdcVlyB/1
  Merge4/1 -> MotCtrlMotCurrAdcVlyC/1
  Bmw5441McuCfgPer3/12(BattVltgSwd1AdcFaild) -> BattVltgSwd1AdcFaild/1
  Bmw5441McuCfgPer3/10(BattVltgAdcFaild) -> BattVltgAdcFaild/1
  Bmw5441McuCfgPer3/13(EcuTAdcFaild) -> EcuTAdcFaild/1
  Bmw5441McuCfgPer3/4(HwTq4RawAdcFaild) -> HwTq4RawAdcFaild/1
  Bmw5441McuCfgPer3/5(HwTq5RawAdcFaild) -> HwTq5RawAdcFaild/1
  Bmw5441McuCfgPer3/1(MotCurrAdcVlyAAdcFaild) -> MotCurrAdcVlyAAdcFaild/1
  Bmw5441McuCfgPer3/2(MotCurrAdcVlyBAdcFaild) -> MotCurrAdcVlyBAdcFaild/1
  Bmw5441McuCfgPer3/3(MotCurrAdcVlyCAdcFaild) -> MotCurrAdcVlyCAdcFaild/1
  Bmw5441McuCfgPer3/6(MotCurrAdcPeakAAdcFaild) -> MotCurrAdcPeakAAdcFaild/1
  Bmw5441McuCfgPer3/7(MotCurrAdcPeakBAdcFaild) -> MotCurrAdcPeakBAdcFaild/1
  Bmw5441McuCfgPer3/8(MotCurrAdcPeakCAdcFaild) -> MotCurrAdcPeakCAdcFaild/1
  Bmw5441McuCfgPer3/9(MotCurrSnsrOffs1AdcFaild) -> MotCurrSnsrOffs1AdcFaild/1
  Bmw5441McuCfgInit2/1(MotCtrlAdc0ScanGroup3Ref0) -> [MotCtrlAdc0ScanGroup3Ref0_init]
  Bmw5441McuCfgInit2/2(MotCtrlMotCurrAdcVlyA) -> [MotCtrlMotCurrAdcVlyA_init]
  Bmw5441McuCfgInit2/3(MotCtrlMotCurrAdcVlyB) -> [MotCtrlMotCurrAdcVlyB_init]
  Bmw5441McuCfgPer1/1(MotCtrlAdc0ScanGroup3Ref0) -> [MotCtrlAdc0ScanGroup3Ref0]
  Bmw5441McuCfgPer1/2(MotCtrlMotCurrAdcVlyA) -> [MotCtrlMotCurrAdcVlyA]
  Bmw5441McuCfgPer1/3(MotCtrlMotCurrAdcVlyB) -> [MotCtrlMotCurrAdcVlyB]
  Bmw5441McuCfgPer1/4(MotCtrlMotCurrAdcVlyC) -> [MotCtrlMotCurrAdcVlyC]
  Bmw5441McuCfgPer1/13(T1Adc) -> [HwTq4RawAdc]
  Bmw5441McuCfgPer1/14(T2Adc) -> [HwTq5RawAdc]
  Bmw5441McuCfgInit2/4(MotCtrlMotCurrAdcVlyC) -> [MotCtrlMotCurrAdcVlyC_init]
  Bmw5441McuCfgInit2/13(HwTq4RawAdc) -> [HwTq4RawAdc_init]
  Bmw5441McuCfgInit2/14(HwTq5RawAdc) -> [HwTq5RawAdc_init]
  Bmw5441McuCfgInit2/5(MotCtrlAdc0ScanGroup3Ref1) -> [MotCtrlAdc0ScanGroup3Ref1_init]
  Bmw5441McuCfgInit2/6(MotCtrlAdc0ScanGroup2Ref0) -> [MotCtrlAdc0ScanGroup2Ref0_init]
  Bmw5441McuCfgInit2/7(MotCtrlMotCurrAdcPeakA) -> [MotCtrlMotCurrAdcPeakA_init]
  Bmw5441McuCfgInit2/8(MotCtrlMotCurrAdcPeakB) -> [MotCtrlMotCurrAdcPeakB_init]
  Bmw5441McuCfgInit2/9(MotCtrlMotCurrAdcPeakC) -> [MotCtrlMotCurrAdcPeakC_init]
  Bmw5441McuCfgInit2/10(MotCtrlMotCurrSnsrOffs1) -> [MotCtrlMotCurrSnsrOffs1_init]
  Bmw5441McuCfgInit2/11(BattVltgAdc) -> [MotCtrlBattVltgAdc_init]
  Bmw5441McuCfgInit2/15(MotCtrlAdc0ScanGroup2Ref1) -> [MotCtrlAdc0ScanGroup2Ref1_init]
  Bmw5441McuCfgInit2/16(MotCtrlAdc0SelfDiag0) -> [MotCtrlAdc0SelfDiag0_init]
  Bmw5441McuCfgInit2/17(MotCtrlAdc0SelfDiag2) -> [MotCtrlAdc0SelfDiag2_init]
  Bmw5441McuCfgInit2/18(MotCtrlAdc0SelfDiag4) -> [MotCtrlAdc0SelfDiag4_init]
  Bmw5441McuCfgPer1/5(MotCtrlAdc0ScanGroup3Ref1) -> [MotCtrlAdc0ScanGroup3Ref1]
  Bmw5441McuCfgPer1/6(MotCtrlAdc0ScanGroup2Ref0) -> [MotCtrlAdc0ScanGroup2Ref0]
  Bmw5441McuCfgPer1/7(MotCtrlMotCurrAdcPeakA) -> [MotCtrlMotCurrAdcPeakA]
  Bmw5441McuCfgPer1/8(MotCtrlMotCurrAdcPeakB) -> [MotCtrlMotCurrAdcPeakB]
  Bmw5441McuCfgPer1/9(MotCtrlMotCurrAdcPeakC) -> [MotCtrlMotCurrAdcPeakC]
  Bmw5441McuCfgPer1/10(MotCtrlMotCurrSnsrOffs1) -> [MotCtrlMotCurrSnsrOffs1]
  Bmw5441McuCfgPer1/11(BattVltgAdc) -> [MotCtrlBattVltgAdc]
  Bmw5441McuCfgPer1/15(MotCtrlAdc0ScanGroup2Ref1) -> [MotCtrlAdc0ScanGroup2Ref1]
  Bmw5441McuCfgPer1/16(MotCtrlAdc0SelfDiag0) -> [MotCtrlAdc0SelfDiag0]
  Bmw5441McuCfgPer1/17(MotCtrlAdc0SelfDiag2) -> [MotCtrlAdc0SelfDiag2]
  Bmw5441McuCfgPer1/18(MotCtrlAdc0SelfDiag4) -> [MotCtrlAdc0SelfDiag4]
  [MotCtrlAdc0ScanGroup3Ref0_init] -> Merge1/1
  [MotCtrlAdc0ScanGroup3Ref0] -> Merge1/2
  [MotCtrlMotCurrAdcVlyA_init] -> Merge2/1
  [MotCtrlMotCurrAdcVlyA] -> Merge2/2
  [MotCtrlMotCurrAdcVlyB_init] -> Merge3/1
  [MotCtrlMotCurrAdcVlyB] -> Merge3/2
  [MotCtrlMotCurrAdcVlyC_init] -> Merge4/1
  [MotCtrlMotCurrAdcVlyC] -> Merge4/2
  [MotCtrlAdc0ScanGroup3Ref1_init] -> Merge26/1
  [MotCtrlAdc0ScanGroup3Ref1] -> Merge26/2
  [MotCtrlAdc0ScanGroup2Ref0_init] -> Merge28/1
  [MotCtrlAdc0ScanGroup2Ref0] -> Merge28/2
  [MotCtrlMotCurrAdcPeakA_init] -> Merge34/1
  [MotCtrlMotCurrAdcPeakA] -> Merge34/2
  [MotCtrlMotCurrAdcPeakB_init] -> Merge35/1
  [MotCtrlMotCurrAdcPeakB] -> Merge35/2
  Merge35/1 -> MotCtrlMotCurrAdcPeakB/1
  Merge26/1 -> MotCtrlAdc0ScanGroup3Ref1/1
  Merge28/1 -> MotCtrlAdc0ScanGroup2Ref0/1
  Merge34/1 -> MotCtrlMotCurrAdcPeakA/1
  [MotCtrlMotCurrAdcPeakC_init] -> Merge36/1
  [MotCtrlMotCurrAdcPeakC] -> Merge36/2
  [MotCtrlMotCurrSnsrOffs1_init] -> Merge37/1
  [MotCtrlMotCurrSnsrOffs1] -> Merge37/2
  [MotCtrlAdc0ScanGroup2Ref1_init] -> Merge38/1
  [MotCtrlAdc0ScanGroup2Ref1] -> Merge38/2
  Merge38/1 -> MotCtrlAdc0ScanGroup2Ref1/1
  Merge36/1 -> MotCtrlMotCurrAdcPeakC/1
  Merge37/1 -> MotCtrlMotCurrSnsrOffs1/1
  Merge5/1 -> MotCtrlAdc0SelfDiag0/1
  Merge9/1 -> MotCtrlAdc0SelfDiag2/1
  Merge10/1 -> MotCtrlAdc0SelfDiag4/1
  [MotCtrlAdc0SelfDiag0_init] -> Merge5/1
  [MotCtrlAdc0SelfDiag0] -> Merge5/2
  [MotCtrlAdc0SelfDiag2_init] -> Merge9/1
  [MotCtrlAdc0SelfDiag2] -> Merge9/2
  [MotCtrlAdc0SelfDiag4_init] -> Merge10/1
  [MotCtrlAdc0SelfDiag4] -> Merge10/2
  Bmw5441McuCfgInit3/2(BattVltgSwd1) -> [BattVltgSwd1_init]
  Bmw5441McuCfgInit3/3(EcuT) -> [EcuT_init]
  Bmw5441McuCfgInit3/1(Adc1ScanGroup3Ref0) -> [Adc1ScanGroup3Ref0_init]
  Bmw5441McuCfgInit3/4(Adc1ScanGroup3Ref1) -> [Adc1ScanGroup3Ref1_init]
  Bmw5441McuCfgInit3/5(Adc1ScanGroup2Ref0) -> [Adc1ScanGroup2Ref0_init]
  Bmw5441McuCfgInit3/6(RvsBattDiagcGndAdc) -> [RvsBattDiagcGndAdc_init]
  Bmw5441McuCfgInit3/7(RvsBattDiagcRtnAdc) -> [RvsBattDiagcRtnAdc_init]
  Bmw5441McuCfgInit3/8(Adc1ScanGroup2Ref1) -> [Adc1ScanGroup2Ref1_init]
  Bmw5441McuCfgInit3/9(Adc1SelfDiag0) -> [Adc1SelfDiag0_init]
  Bmw5441McuCfgInit3/10(Adc1SelfDiag2) -> [Adc1SelfDiag2_init]
  Bmw5441McuCfgInit3/11(Adc1SelfDiag4) -> [Adc1SelfDiag4_init]
  Bmw5441McuCfgPer2/1(Adc1ScanGroup3Ref0) -> [Adc1ScanGroup3Ref0]
  Bmw5441McuCfgPer2/2(BattVltgSwd1) -> [BattVltgSwd1]
  Bmw5441McuCfgPer2/3(EcuT) -> [EcuT]
  Bmw5441McuCfgPer2/4(Adc1ScanGroup3Ref1) -> [Adc1ScanGroup3Ref1]
  Bmw5441McuCfgPer2/5(Adc1ScanGroup2Ref0) -> [Adc1ScanGroup2Ref0]
  Bmw5441McuCfgPer2/6(RvsBattDiagcGndAdc) -> [RvsBattDiagcGndAdc]
  Bmw5441McuCfgPer2/7(RvsBattDiagcRtnAdc) -> [RvsBattDiagcRtnAdc]
  Bmw5441McuCfgPer2/8(Adc1ScanGroup2Ref1) -> [Adc1ScanGroup2Ref1]
  Bmw5441McuCfgPer2/9(Adc1SelfDiag0) -> [Adc1SelfDiag0]
  Bmw5441McuCfgPer2/10(Adc1SelfDiag2) -> [Adc1SelfDiag2]
  Bmw5441McuCfgPer2/11(Adc1SelfDiag4) -> [Adc1SelfDiag4]
  Merge6/1 -> Adc1ScanGroup3Ref0/1
  Merge7/1 -> BattVltgSwd1/1
  Merge12/1 -> EcuT/1
  Merge21/1 -> Adc1ScanGroup3Ref1/1
  [Adc1ScanGroup3Ref0_init] -> Merge6/1
  [Adc1ScanGroup3Ref0] -> Merge6/2
  [BattVltgSwd1_init] -> Merge7/1
  [BattVltgSwd1] -> Merge7/2
  [EcuT_init] -> Merge12/1
  [EcuT] -> Merge12/2
  [Adc1ScanGroup3Ref1_init] -> Merge21/1
  [Adc1ScanGroup3Ref1] -> Merge21/2
  [Adc1ScanGroup2Ref0_init] -> Merge8/1
  [Adc1ScanGroup2Ref0] -> Merge8/2
  [RvsBattDiagcGndAdc_init] -> Merge11/1
  [RvsBattDiagcGndAdc] -> Merge11/2
  [RvsBattDiagcRtnAdc_init] -> Merge13/1
  [RvsBattDiagcRtnAdc] -> Merge13/2
  [Adc1ScanGroup2Ref1_init] -> Merge14/1
  [Adc1ScanGroup2Ref1] -> Merge14/2
  Merge14/1 -> Adc1ScanGroup2Ref1/1
  Merge8/1 -> Adc1ScanGroup2Ref0/1
  Merge11/1 -> RvsBattDiagcGndAdc/1
  Merge13/1 -> RvsBattDiagcRtnAdc/1
  [Adc1SelfDiag0_init] -> Merge15/1
  [Adc1SelfDiag0] -> Merge15/2
  [Adc1SelfDiag2_init] -> Merge16/1
  [Adc1SelfDiag2] -> Merge16/2
  [Adc1SelfDiag4_init] -> Merge17/1
  [Adc1SelfDiag4] -> Merge17/2
  Merge17/1 -> Adc1SelfDiag4/1
  Merge15/1 -> Adc1SelfDiag0/1
  Merge16/1 -> Adc1SelfDiag2/1
  Merge18/1 -> MotCtrlHwTq4RawAdc/1
  Merge19/1 -> MotCtrlHwTq5RawAdc/1
  [MotCtrlBattVltgAdc_init] -> Merge20/1
  [MotCtrlBattVltgAdc] -> Merge20/2
  Merge20/1 -> MotCtrlBattVltgAdc/1
  [HwTq4RawAdc_init] -> Merge18/1
  [HwTq4RawAdc] -> Merge18/2
  [HwTq5RawAdc_init] -> Merge19/1
  [HwTq5RawAdc] -> Merge19/2
  Bmw5441McuCfgInit2/12(BattRtnCurrAdc) -> [MotCtrlBattRtnCurrAdc_init]
  Bmw5441McuCfgPer1/12(BattRtnCurrAdc) -> [MotCtrlBattRtnCurrAdc]
  [MotCtrlBattRtnCurrAdc_init] -> Merge22/1
  [MotCtrlBattRtnCurrAdc] -> Merge22/2
  Merge22/1 -> MotCtrlBattRtnCurrAdc/1
  Bmw5441McuCfgPer3/14(RvsBattDiagcGndAdcFaild) -> RvsBattDiagcGndAdcFaild/1
  Bmw5441McuCfgPer3/15(RvsBattDiagcRtnAdcFaild) -> RvsBattDiagcRtnAdcFaild/1
  Bmw5441McuCfgPer3/11(BattRtnCurrAdcFaild) -> BattRtnCurrAdcFaild/1
  Bmw5441McuCfgPer3/16(MotDrvr1IninTestCmpl) -> MotDrvr1IninTestCmpl/1

== system CM020A_Bmw5441McuCfg/CopyRight2 ==

== system CM020A_Bmw5441McuCfg/Bmw5441McuCfg/Bmw5441McuCfgInit1 ==
  function : TriggerPort  TriggerType=function-call
  CopyRight2 : Subsystem  Description=|  mask(Copyright Information){none=on}
      | Copyright info block.                                               
      |                                                                     
      | Place copyright information at the top of every subsystem in design.
      mask prompts: none "No parameters"
      mask help: Place copyright information at the top of every subsystem in design.
      mask Display:
      | NxtrConf = 'Nexteer Confidential';
      | 
      | sys = bdroot; %handle for the current model ("system")
      | first = get_param(sys,'Created');
      | first = first(end-3:end);  %year is last four digits
      | 
      | last = get_param(sys,'LastModifiedDate');
      | if isempty(last)
      |     last = datestr(now,'yyyy');
      | else
      |     last = last(end-3:end);
      | end
      | 
      | if strcmp(first,last)
      |     fprintf('%s -- Copyright %s Nexteer',NxtrConf,first)
      | else
      |     fprintf('%s -- %s%s- %s Nexteer',NxtrConf,char(169),first,last)
      | end
  Do Not Code : Subsystem
  Register Initialization : Subsystem  Priority=10
      settings: AttributesFormatString=Priority: %<Priority>

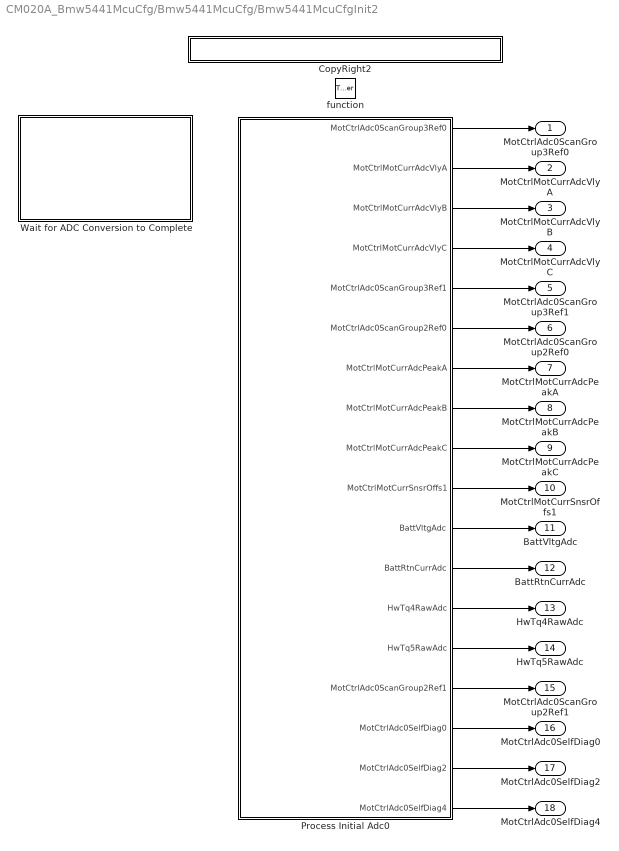
== system CM020A_Bmw5441McuCfg/Bmw5441McuCfg/Bmw5441McuCfgInit2 ==
  function : TriggerPort  TriggerType=function-call
  CopyRight2 : Subsystem  Description=|  mask(Copyright Information){none=on}
      | Copyright info block.                                               
      |                                                                     
      | Place copyright information at the top of every subsystem in design.
      mask prompts: none "No parameters"
      mask help: Place copyright information at the top of every subsystem in design.
      mask Display:
      | NxtrConf = 'Nexteer Confidential';
      | 
      | sys = bdroot; %handle for the current model ("system")
      | first = get_param(sys,'Created');
      | first = first(end-3:end);  %year is last four digits
      | 
      | last = get_param(sys,'LastModifiedDate');
      | if isempty(last)
      |     last = datestr(now,'yyyy');
      | else
      |     last = last(end-3:end);
      | end
      | 
      | if strcmp(first,last)
      |     fprintf('%s -- Copyright %s Nexteer',NxtrConf,first)
      | else
      |     fprintf('%s -- %s%s- %s Nexteer',NxtrConf,char(169),first,last)
      | end
  Process Initial Adc0 : Subsystem  RequirementInfo="{'linktype_rmi_doors' '0000c472 (/ESG Group/FDD Module Requirements/EA4 Specific/CM300A_Adc0CfgAndUse)' '#CM300A_76' 'true' 'REQ: CM300A_76' '' ; 'linktype_rmi_doors' '0000c472 (/ESG Group/FDD Module Requirements/EA4 Specific/CM300A_Adc0CfgAndUse)' '#CM300A_95' 'true' 'REQ:  CM300A_95' '' } %GIDa_d862d82c_969a_40be_9cba_5dad28e4f649"  Priority=20
      settings: AttributesFormatString=Priority: %<Priority>
  Wait for ADC Conversion to Complete : Subsystem  Priority=10
      settings: AttributesFormatString=Priority: %<Priority>
  MotCtrlAdc0ScanGroup3Ref0 : Outport
  MotCtrlMotCurrAdcVlyA : Outport  Port=2
  MotCtrlMotCurrAdcVlyB : Outport  Port=3
  MotCtrlMotCurrAdcVlyC : Outport  Port=4
  MotCtrlAdc0ScanGroup3Ref1 : Outport  Port=5
  MotCtrlAdc0ScanGroup2Ref0 : Outport  Port=6
  MotCtrlMotCurrAdcPeakA : Outport  Port=7
  MotCtrlMotCurrAdcPeakB : Outport  Port=8
  MotCtrlMotCurrAdcPeakC : Outport  Port=9
  MotCtrlMotCurrSnsrOffs1 : Outport  Port=10
  BattVltgAdc : Outport  Port=11
  BattRtnCurrAdc : Outport  Port=12
  HwTq4RawAdc : Outport  Port=13
  HwTq5RawAdc : Outport  Port=14
  MotCtrlAdc0ScanGroup2Ref1 : Outport  Port=15
  MotCtrlAdc0SelfDiag0 : Outport  Port=16
  MotCtrlAdc0SelfDiag2 : Outport  Port=17
  MotCtrlAdc0SelfDiag4 : Outport  Port=18
  wires:
  Process Initial Adc0/1(MotCtrlAdc0ScanGroup3Ref0) -> MotCtrlAdc0ScanGroup3Ref0/1
  Process Initial Adc0/2(MotCtrlMotCurrAdcVlyA) -> MotCtrlMotCurrAdcVlyA/1
  Process Initial Adc0/3(MotCtrlMotCurrAdcVlyB) -> MotCtrlMotCurrAdcVlyB/1
  Process Initial Adc0/4(MotCtrlMotCurrAdcVlyC) -> MotCtrlMotCurrAdcVlyC/1
  Process Initial Adc0/5(MotCtrlAdc0ScanGroup3Ref1) -> MotCtrlAdc0ScanGroup3Ref1/1
  Process Initial Adc0/6(MotCtrlAdc0ScanGroup2Ref0) -> MotCtrlAdc0ScanGroup2Ref0/1
  Process Initial Adc0/7(MotCtrlMotCurrAdcPeakA) -> MotCtrlMotCurrAdcPeakA/1
  Process Initial Adc0/8(MotCtrlMotCurrAdcPeakB) -> MotCtrlMotCurrAdcPeakB/1
  Process Initial Adc0/9(MotCtrlMotCurrAdcPeakC) -> MotCtrlMotCurrAdcPeakC/1
  Process Initial Adc0/10(MotCtrlMotCurrSnsrOffs1) -> MotCtrlMotCurrSnsrOffs1/1
  Process Initial Adc0/16(MotCtrlAdc0SelfDiag0) -> MotCtrlAdc0SelfDiag0/1
  Process Initial Adc0/17(MotCtrlAdc0SelfDiag2) -> MotCtrlAdc0SelfDiag2/1
  Process Initial Adc0/18(MotCtrlAdc0SelfDiag4) -> MotCtrlAdc0SelfDiag4/1
  Process Initial Adc0/13(HwTq4RawAdc) -> HwTq4RawAdc/1
  Process Initial Adc0/14(HwTq5RawAdc) -> HwTq5RawAdc/1
  Process Initial Adc0/11(BattVltgAdc) -> BattVltgAdc/1
  Process Initial Adc0/15(MotCtrlAdc0ScanGroup2Ref1) -> MotCtrlAdc0ScanGroup2Ref1/1
  Process Initial Adc0/12(BattRtnCurrAdc) -> BattRtnCurrAdc/1

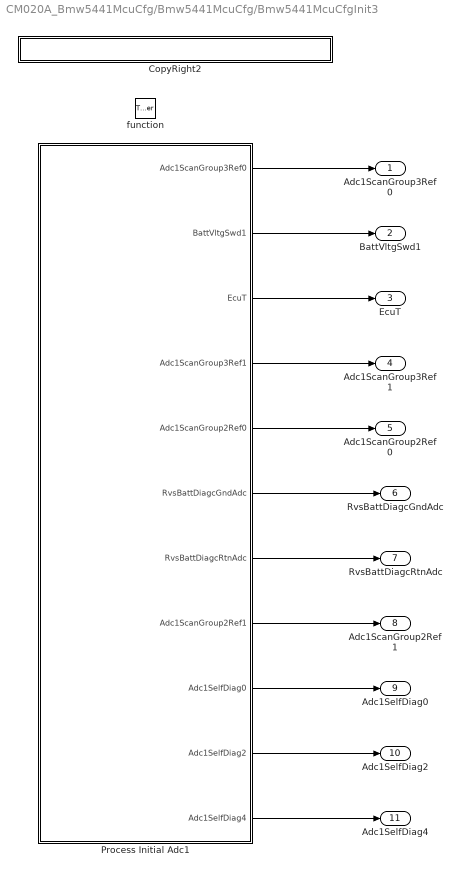
== system CM020A_Bmw5441McuCfg/Bmw5441McuCfg/Bmw5441McuCfgInit3 ==
  function : TriggerPort  TriggerType=function-call
  CopyRight2 : Subsystem  Description=|  mask(Copyright Information){none=on}
      | Copyright info block.                                               
      |                                                                     
      | Place copyright information at the top of every subsystem in design.
      mask prompts: none "No parameters"
      mask help: Place copyright information at the top of every subsystem in design.
      mask Display:
      | NxtrConf = 'Nexteer Confidential';
      | 
      | sys = bdroot; %handle for the current model ("system")
      | first = get_param(sys,'Created');
      | first = first(end-3:end);  %year is last four digits
      | 
      | last = get_param(sys,'LastModifiedDate');
      | if isempty(last)
      |     last = datestr(now,'yyyy');
      | else
      |     last = last(end-3:end);
      | end
      | 
      | if strcmp(first,last)
      |     fprintf('%s -- Copyright %s Nexteer',NxtrConf,first)
      | else
      |     fprintf('%s -- %s%s- %s Nexteer',NxtrConf,char(169),first,last)
      | end
  Process Initial Adc1 : Subsystem  RequirementInfo="{'linktype_rmi_doors' '0000c475 (/ESG Group/FDD Module Requirements/EA4 Specific/CM320A_Adc1CfgAndUse)' '#CM320A_92' 'true' 'REQ:  CM320A_92' '' ; 'linktype_rmi_doors' '0000c475 (/ESG Group/FDD Module Requirements/EA4 Specific/CM320A_Adc1CfgAndUse)' '#CM320A_76' 'true' 'REQ:  CM320A_76' '' } %GIDa_376048c3_94d2_40f9_9974_227dea3c5b4f"  Priority=40
      settings: AttributesFormatString=Priority: %<Priority>
  Adc1ScanGroup3Ref0 : Outport
  BattVltgSwd1 : Outport  Port=2
  EcuT : Outport  Port=3
  Adc1ScanGroup3Ref1 : Outport  Port=4
  Adc1ScanGroup2Ref0 : Outport  Port=5
  RvsBattDiagcGndAdc : Outport  Port=6
  RvsBattDiagcRtnAdc : Outport  Port=7
  Adc1ScanGroup2Ref1 : Outport  Port=8
  Adc1SelfDiag0 : Outport  Port=9
  Adc1SelfDiag2 : Outport  Port=10
  Adc1SelfDiag4 : Outport  Port=11
  wires:
  Process Initial Adc1/1(Adc1ScanGroup3Ref0) -> Adc1ScanGroup3Ref0/1
  Process Initial Adc1/2(BattVltgSwd1) -> BattVltgSwd1/1
  Process Initial Adc1/3(EcuT) -> EcuT/1
  Process Initial Adc1/4(Adc1ScanGroup3Ref1) -> Adc1ScanGroup3Ref1/1
  Process Initial Adc1/5(Adc1ScanGroup2Ref0) -> Adc1ScanGroup2Ref0/1
  Process Initial Adc1/6(RvsBattDiagcGndAdc) -> RvsBattDiagcGndAdc/1
  Process Initial Adc1/9(Adc1SelfDiag0) -> Adc1SelfDiag0/1
  Process Initial Adc1/10(Adc1SelfDiag2) -> Adc1SelfDiag2/1
  Process Initial Adc1/11(Adc1SelfDiag4) -> Adc1SelfDiag4/1
  Process Initial Adc1/7(RvsBattDiagcRtnAdc) -> RvsBattDiagcRtnAdc/1
  Process Initial Adc1/8(Adc1ScanGroup2Ref1) -> Adc1ScanGroup2Ref1/1

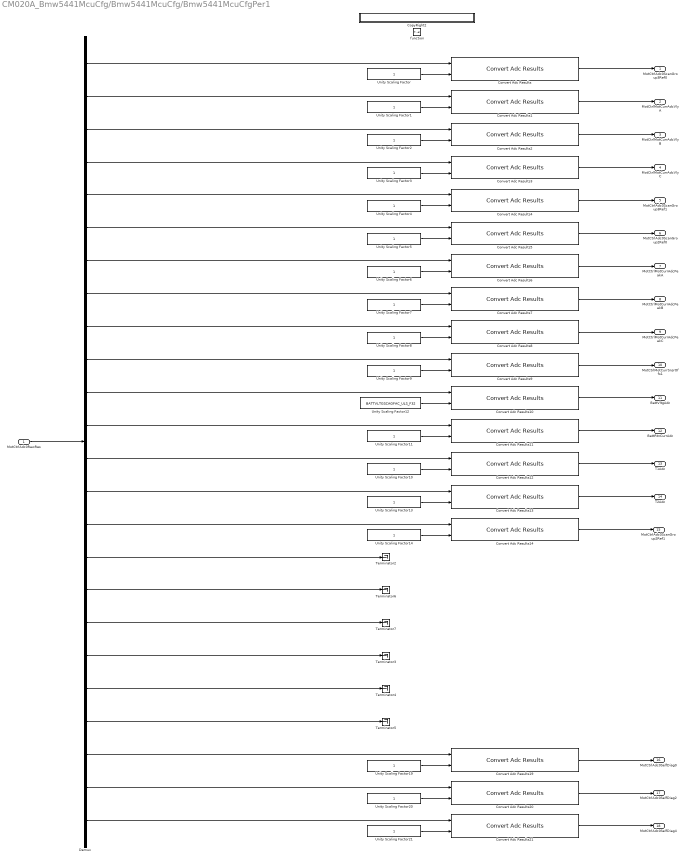
== system CM020A_Bmw5441McuCfg/Bmw5441McuCfg/Bmw5441McuCfgPer1 ==
  MotCtrlAdc0RawRes : Inport
  function : TriggerPort  TriggerType=function-call
  Convert Adc Results{,1..14,19..21} (18 alike) : CM020A_Bmw5441McuCfg_ModelLibrary/Convert Adc Results
  CopyRight2 : Subsystem  Description=|  mask(Copyright Information){none=on}
      | Copyright info block.                                               
      |                                                                     
      | Place copyright information at the top of every subsystem in design.
      mask prompts: none "No parameters"
      mask help: Place copyright information at the top of every subsystem in design.
      mask Display:
      | NxtrConf = 'Nexteer Confidential';
      | 
      | sys = bdroot; %handle for the current model ("system")
      | first = get_param(sys,'Created');
      | first = first(end-3:end);  %year is last four digits
      | 
      | last = get_param(sys,'LastModifiedDate');
      | if isempty(last)
      |     last = datestr(now,'yyyy');
      | else
      |     last = last(end-3:end);
      | end
      | 
      | if strcmp(first,last)
      |     fprintf('%s -- Copyright %s Nexteer',NxtrConf,first)
      | else
      |     fprintf('%s -- %s%s- %s Nexteer',NxtrConf,char(169),first,last)
      | end
  Demux : Demux  Outputs=24
  Terminator{2..7} (6 alike) : Terminator
  Unity Scaling Factor{,1..11,13..14,19..21} (17 alike) : Constant  OutDataTypeStr=single
  Unity Scaling Factor12 : Constant  Value=BATTVLTGSCAGFAC_ULS_F32  OutDataTypeStr=single
  MotCtrlAdc0ScanGroup3Ref0 : Outport
  MotCtrlMotCurrAdcVlyA : Outport  Port=2
  MotCtrlMotCurrAdcVlyB : Outport  Port=3
  MotCtrlMotCurrAdcVlyC : Outport  Port=4
  MotCtrlAdc0ScanGroup3Ref1 : Outport  Port=5
  MotCtrlAdc0ScanGroup2Ref0 : Outport  Port=6
  MotCtrlMotCurrAdcPeakA : Outport  Port=7
  MotCtrlMotCurrAdcPeakB : Outport  Port=8
  MotCtrlMotCurrAdcPeakC : Outport  Port=9
  MotCtrlMotCurrSnsrOffs1 : Outport  Port=10
  BattVltgAdc : Outport  Port=11
  BattRtnCurrAdc : Outport  Port=12
  T1Adc : Outport  Port=13
  T2Adc : Outport  Port=14
  MotCtrlAdc0ScanGroup2Ref1 : Outport  Port=15
  MotCtrlAdc0SelfDiag0 : Outport  Port=16
  MotCtrlAdc0SelfDiag2 : Outport  Port=17
  MotCtrlAdc0SelfDiag4 : Outport  Port=18
  wires:
  MotCtrlAdc0RawRes/1 -> Demux/1
  Unity Scaling Factor/1 -> Convert Adc Results/2
  Unity Scaling Factor1/1 -> Convert Adc Results1/2
  Unity Scaling Factor2/1 -> Convert Adc Results2/2
  Unity Scaling Factor3/1 -> Convert Adc Results3/2
  Unity Scaling Factor4/1 -> Convert Adc Results4/2
  Unity Scaling Factor5/1 -> Convert Adc Results5/2
  Unity Scaling Factor6/1 -> Convert Adc Results6/2
  Unity Scaling Factor7/1 -> Convert Adc Results7/2
  Unity Scaling Factor8/1 -> Convert Adc Results8/2
  Unity Scaling Factor19/1 -> Convert Adc Results19/2
  Unity Scaling Factor20/1 -> Convert Adc Results20/2
  Unity Scaling Factor21/1 -> Convert Adc Results21/2
  Demux/4 -> Convert Adc Results3/1
  Demux/24 -> Convert Adc Results21/1
  Demux/23 -> Convert Adc Results20/1
  Demux/22 -> Convert Adc Results19/1
  Demux/21 -> Terminator5/1
  Demux/19 -> Terminator3/1
  Demux/20 -> Terminator4/1
  Demux/9 -> Convert Adc Results8/1
  Demux/7 -> Convert Adc Results6/1
  Demux/8 -> Convert Adc Results7/1
  Demux/5 -> Convert Adc Results4/1
  Demux/6 -> Convert Adc Results5/1
  Unity Scaling Factor9/1 -> Convert Adc Results9/2
  Unity Scaling Factor11/1 -> Convert Adc Results11/2
  Unity Scaling Factor13/1 -> Convert Adc Results13/2
  Demux/10 -> Convert Adc Results9/1
  Demux/15 -> Convert Adc Results14/1
  Demux/13 -> Convert Adc Results12/1
  Demux/14 -> Convert Adc Results13/1
  Demux/11 -> Convert Adc Results10/1
  Demux/12 -> Convert Adc Results11/1
  Demux/18 -> Terminator7/1
  Demux/16 -> Terminator2/1
  Demux/17 -> Terminator6/1
  Demux/1 -> Convert Adc Results/1
  Demux/2 -> Convert Adc Results1/1
  Demux/3 -> Convert Adc Results2/1
  Convert Adc Results/1 -> MotCtrlAdc0ScanGroup3Ref0/1
  Convert Adc Results19/1 -> MotCtrlAdc0SelfDiag0/1
  Convert Adc Results21/1 -> MotCtrlAdc0SelfDiag4/1
  Convert Adc Results20/1 -> MotCtrlAdc0SelfDiag2/1
  Convert Adc Results1/1 -> MotCtrlMotCurrAdcVlyA/1
  Convert Adc Results2/1 -> MotCtrlMotCurrAdcVlyB/1
  Convert Adc Results3/1 -> MotCtrlMotCurrAdcVlyC/1
  Convert Adc Results4/1 -> MotCtrlAdc0ScanGroup3Ref1/1
  Convert Adc Results5/1 -> MotCtrlAdc0ScanGroup2Ref0/1
  Convert Adc Results6/1 -> MotCtrlMotCurrAdcPeakA/1
  Convert Adc Results7/1 -> MotCtrlMotCurrAdcPeakB/1
  Convert Adc Results8/1 -> MotCtrlMotCurrAdcPeakC/1
  Convert Adc Results9/1 -> MotCtrlMotCurrSnsrOffs1/1
  Convert Adc Results10/1 -> BattVltgAdc/1
  Convert Adc Results11/1 -> BattRtnCurrAdc/1
  Convert Adc Results12/1 -> T1Adc/1
  Unity Scaling Factor14/1 -> Convert Adc Results14/2
  Convert Adc Results14/1 -> MotCtrlAdc0ScanGroup2Ref1/1
  Convert Adc Results13/1 -> T2Adc/1
  Unity Scaling Factor10/1 -> Convert Adc Results12/2
  Unity Scaling Factor12/1 -> Convert Adc Results10/2
